simulink model "Glucose_Insulin_Model"  (R2024b)
settings: Solver=ode1  StartTime=0.0  StopTime=5  FixedStep=0.01  RelTol=1e-3
settings Model: Creator=nafis  LastModifiedBy=nafis
settings SolverCC: DateTimeAtSimulationTimeZero=[]

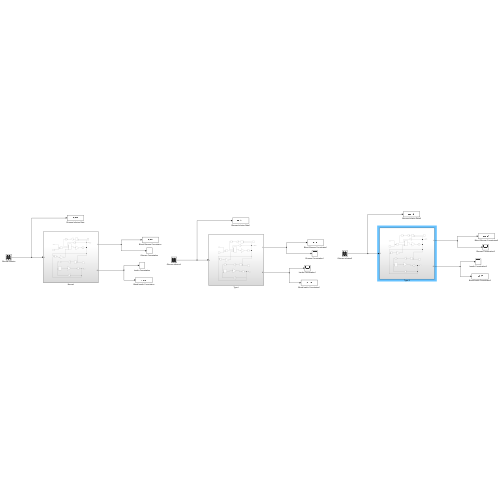
[thumbnail: Simulink's stored preview of the top-level diagram]
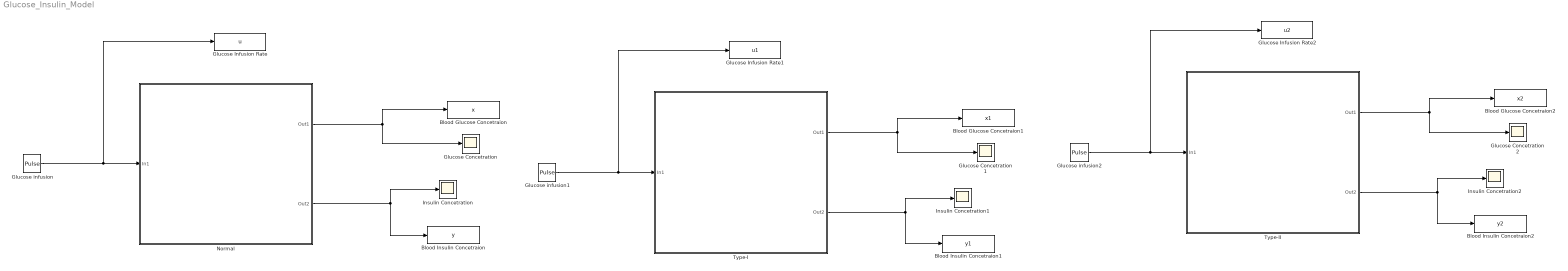
== system Glucose_Insulin_Model ==
  Blood Glucose Concetraion : ToWorkspace  VariableName=x  SaveFormat=Timeseries  SampleTime=-1
  Blood Glucose Concetraion1 : ToWorkspace  VariableName=x1  SaveFormat=Timeseries  SampleTime=-1
  Blood Glucose Concetraion2 : ToWorkspace  VariableName=x2  SaveFormat=Timeseries  SampleTime=-1
  Blood Insulin Concetraion : ToWorkspace  VariableName=y  SaveFormat=Timeseries  SampleTime=-1
  Blood Insulin Concetraion1 : ToWorkspace  VariableName=y1  SaveFormat=Timeseries  SampleTime=-1
  Blood Insulin Concetraion2 : ToWorkspace  VariableName=y2  SaveFormat=Timeseries  SampleTime=-1
  Glucose Concetration : Scope
  Glucose Concetration1 : Scope
  Glucose Concetration2 : Scope
  Glucose Infusion Rate : ToWorkspace  VariableName=u  SaveFormat=Timeseries  SampleTime=-1
  Glucose Infusion Rate1 : ToWorkspace  VariableName=u1  SaveFormat=Timeseries  SampleTime=-1
  Glucose Infusion Rate2 : ToWorkspace  VariableName=u2  SaveFormat=Timeseries  SampleTime=-1
  Glucose infusion : DiscretePulseGenerator  PulseType=Time based  Amplitude=100000  Period=5  PulseWidth=5  PhaseDelay=0.5
  Glucose infusion1 : DiscretePulseGenerator  PulseType=Time based  Amplitude=100000  Period=5  PulseWidth=5  PhaseDelay=0.5
  Glucose infusion2 : DiscretePulseGenerator  PulseType=Time based  Amplitude=100000  Period=5  PulseWidth=5  PhaseDelay=0.5
  Insulin Concetration : Scope
  Insulin Concetration1 : Scope
  Insulin Concetration2 : Scope
  Normal : Subsystem
  Type-I : Subsystem
  Type-II : Subsystem
  wires:
  Glucose infusion/1 -> Glucose Infusion Rate/1, Normal/1(In1)
  Normal/2(Out2) -> Blood Insulin Concetraion/1, Insulin Concetration/1
  Normal/1(Out1) -> Blood Glucose Concetraion/1, Glucose Concetration/1
  Type-I/2(Out2) -> Blood Insulin Concetraion1/1, Insulin Concetration1/1
  Glucose infusion1/1 -> Glucose Infusion Rate1/1, Type-I/1(In1)
  Type-I/1(Out1) -> Blood Glucose Concetraion1/1, Glucose Concetration1/1
  Type-II/2(Out2) -> Blood Insulin Concetraion2/1, Insulin Concetration2/1
  Glucose infusion2/1 -> Glucose Infusion Rate2/1, Type-II/1(In1)
  Type-II/1(Out1) -> Blood Glucose Concetraion2/1, Glucose Concetration2/1

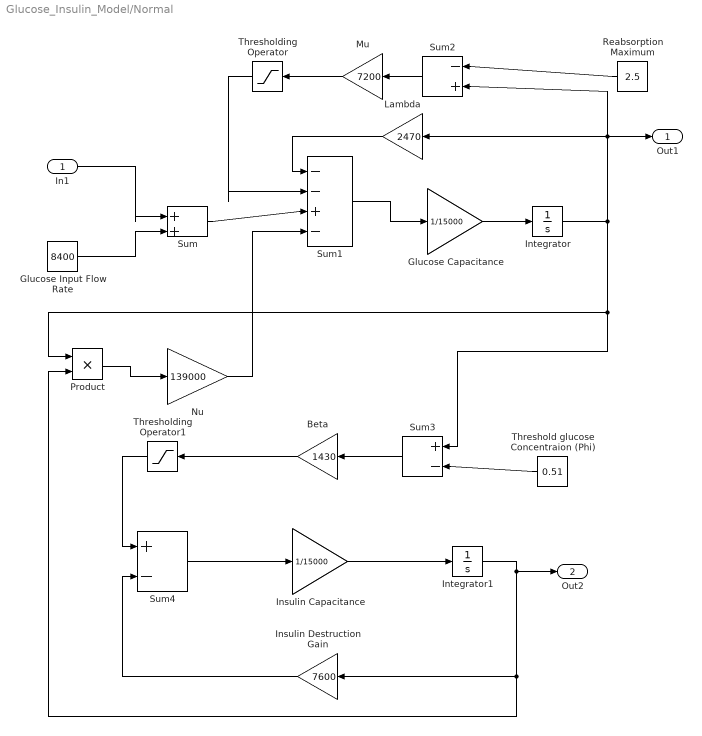
== system Glucose_Insulin_Model/Normal ==
  In1 : Inport
  Beta : Gain  Gain=1430
  Glucose Capacitance : Gain  Gain=1/15000
  Glucose Input Flow Rate : Constant  Value=8400
  Insulin Capacitance : Gain  Gain=1/15000
  Insulin Destruction Gain : Gain  Gain=7600
  Integrator : Integrator  InitialCondition=0.81
  Integrator1 : Integrator  InitialCondition=0.055
  Lambda : Gain  Gain=2470
  Mu : Gain  Gain=7200
  Nu : Gain  Gain=139000
  Product : Product
  Reabsorption Maximum : Constant  Value=2.5
  Sum : Sum  Inputs=|++
  Sum1 : Sum  Inputs=|--+-
  Sum2 : Sum  Inputs=|-+
  Sum3 : Sum  Inputs=|+-
  Sum4 : Sum  Inputs=|+-
  Threshold glucose Concentraion (Phi) : Constant  Value=0.51
  Thresholding Operator : Saturate  UpperLimit=100000  LowerLimit=0  LinearizeAsGain=off
  Thresholding Operator1 : Saturate  UpperLimit=100000  LowerLimit=0
  Out1 : Outport
  Out2 : Outport  Port=2
  wires:
  Glucose Input Flow Rate/1 -> Sum/2
  In1/1 -> Sum/1
  Sum/1 -> Sum1/3
  Thresholding Operator/1 -> Sum1/2
  Mu/1 -> Thresholding Operator/1
  Sum2/1 -> Mu/1
  Reabsorption Maximum/1 -> Sum2/1
  Lambda/1 -> Sum1/1
  Sum1/1 -> Glucose Capacitance/1
  Glucose Capacitance/1 -> Integrator/1
  Integrator/1 -> Product/1, Sum3/1, Lambda/1, Sum2/2, Out1/1
  Product/1 -> Nu/1
  Threshold glucose Concentraion (Phi)/1 -> Sum3/2
  Sum3/1 -> Beta/1
  Beta/1 -> Thresholding Operator1/1
  Thresholding Operator1/1 -> Sum4/1
  Sum4/1 -> Insulin Capacitance/1
  Insulin Capacitance/1 -> Integrator1/1
  Integrator1/1 -> Insulin Destruction Gain/1, Product/2, Out2/1
  Insulin Destruction Gain/1 -> Sum4/2
  Nu/1 -> Sum1/4

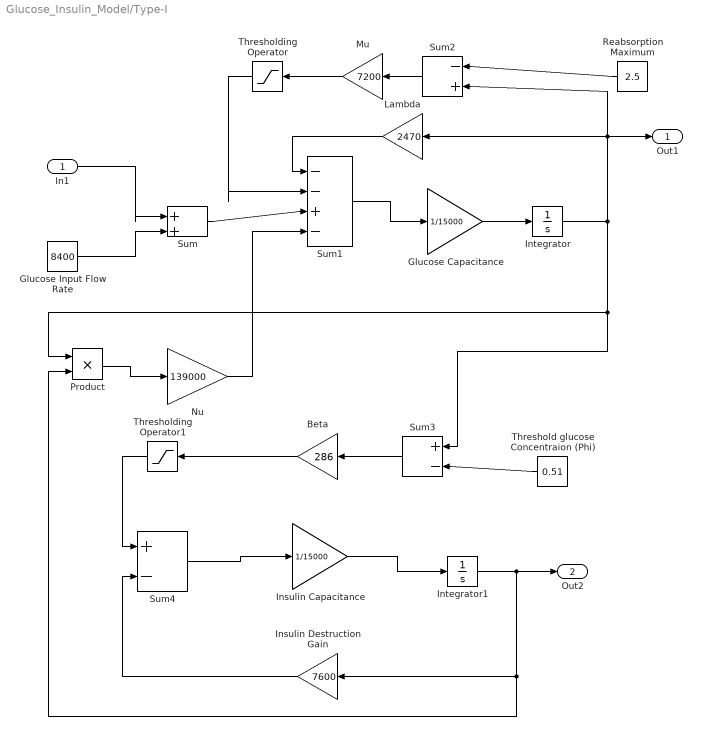
== system Glucose_Insulin_Model/Type-I ==
  In1 : Inport
  Beta : Gain  Gain=286
  Glucose Capacitance : Gain  Gain=1/15000
  Glucose Input Flow Rate : Constant  Value=8400
  Insulin Capacitance : Gain  Gain=1/15000
  Insulin Destruction Gain : Gain  Gain=7600
  Integrator : Integrator  InitialCondition=0.81
  Integrator1 : Integrator  InitialCondition=0.055
  Lambda : Gain  Gain=2470
  Mu : Gain  Gain=7200
  Nu : Gain  Gain=139000
  Product : Product
  Reabsorption Maximum : Constant  Value=2.5
  Sum : Sum  Inputs=|++
  Sum1 : Sum  Inputs=|--+-
  Sum2 : Sum  Inputs=|-+
  Sum3 : Sum  Inputs=|+-
  Sum4 : Sum  Inputs=|+-
  Threshold glucose Concentraion (Phi) : Constant  Value=0.51
  Thresholding Operator : Saturate  UpperLimit=100000  LowerLimit=0
  Thresholding Operator1 : Saturate  UpperLimit=100000  LowerLimit=0
  Out1 : Outport
  Out2 : Outport  Port=2
  wires:
  Glucose Input Flow Rate/1 -> Sum/2
  In1/1 -> Sum/1
  Sum/1 -> Sum1/3
  Thresholding Operator/1 -> Sum1/2
  Mu/1 -> Thresholding Operator/1
  Sum2/1 -> Mu/1
  Reabsorption Maximum/1 -> Sum2/1
  Lambda/1 -> Sum1/1
  Sum1/1 -> Glucose Capacitance/1
  Glucose Capacitance/1 -> Integrator/1
  Integrator/1 -> Product/1, Sum3/1, Lambda/1, Sum2/2, Out1/1
  Product/1 -> Nu/1
  Threshold glucose Concentraion (Phi)/1 -> Sum3/2
  Sum3/1 -> Beta/1
  Beta/1 -> Thresholding Operator1/1
  Thresholding Operator1/1 -> Sum4/1
  Sum4/1 -> Insulin Capacitance/1
  Insulin Capacitance/1 -> Integrator1/1
  Integrator1/1 -> Insulin Destruction Gain/1, Product/2, Out2/1
  Insulin Destruction Gain/1 -> Sum4/2
  Nu/1 -> Sum1/4

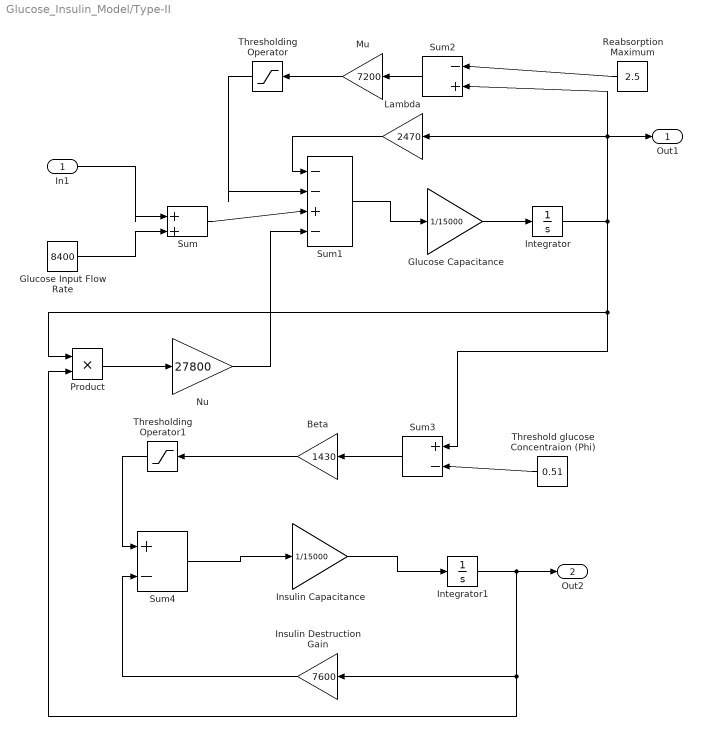
== system Glucose_Insulin_Model/Type-II ==
  In1 : Inport
  Beta : Gain  Gain=1430
  Glucose Capacitance : Gain  Gain=1/15000
  Glucose Input Flow Rate : Constant  Value=8400
  Insulin Capacitance : Gain  Gain=1/15000
  Insulin Destruction Gain : Gain  Gain=7600
  Integrator : Integrator  InitialCondition=0.81
  Integrator1 : Integrator  InitialCondition=0.055
  Lambda : Gain  Gain=2470
  Mu : Gain  Gain=7200
  Nu : Gain  Gain=27800
  Product : Product
  Reabsorption Maximum : Constant  Value=2.5
  Sum : Sum  Inputs=|++
  Sum1 : Sum  Inputs=|--+-
  Sum2 : Sum  Inputs=|-+
  Sum3 : Sum  Inputs=|+-
  Sum4 : Sum  Inputs=|+-
  Threshold glucose Concentraion (Phi) : Constant  Value=0.51
  Thresholding Operator : Saturate  UpperLimit=100000  LowerLimit=0
  Thresholding Operator1 : Saturate  UpperLimit=100000  LowerLimit=0
  Out1 : Outport
  Out2 : Outport  Port=2
  wires:
  Glucose Input Flow Rate/1 -> Sum/2
  In1/1 -> Sum/1
  Sum/1 -> Sum1/3
  Thresholding Operator/1 -> Sum1/2
  Mu/1 -> Thresholding Operator/1
  Sum2/1 -> Mu/1
  Reabsorption Maximum/1 -> Sum2/1
  Lambda/1 -> Sum1/1
  Sum1/1 -> Glucose Capacitance/1
  Glucose Capacitance/1 -> Integrator/1
  Integrator/1 -> Product/1, Sum3/1, Lambda/1, Sum2/2, Out1/1
  Product/1 -> Nu/1
  Threshold glucose Concentraion (Phi)/1 -> Sum3/2
  Sum3/1 -> Beta/1
  Beta/1 -> Thresholding Operator1/1
  Thresholding Operator1/1 -> Sum4/1
  Sum4/1 -> Insulin Capacitance/1
  Insulin Capacitance/1 -> Integrator1/1
  Integrator1/1 -> Insulin Destruction Gain/1, Product/2, Out2/1
  Insulin Destruction Gain/1 -> Sum4/2
  Nu/1 -> Sum1/4
